simulink model "IFSSIM_Powertrain"  (R2025b)
settings: Solver=ode1  StartTime=0  StopTime=inf  FixedStep=0.0010416666666666671  RelTol=1e-3
undefined symbols (not defined in the file or in its folder): battery_builder_rtmsupport, gcbh, IFSSIM_eta, IFSSIM_gr, IFSSIM_Ipk, IFSSIM_Pmax, IFSSIM_Preg, IFSSIM_Tmax, IFSSIM_Treg, IFSSIM_Ts, IFSSIM_wregen
libraries: IFSSIM_Battery_6p19s5m1x_lib x5, fl_lib x3, nesl_utility x3
settings Model: Creator=raulmoran  LastModifiedBy=raulmoran

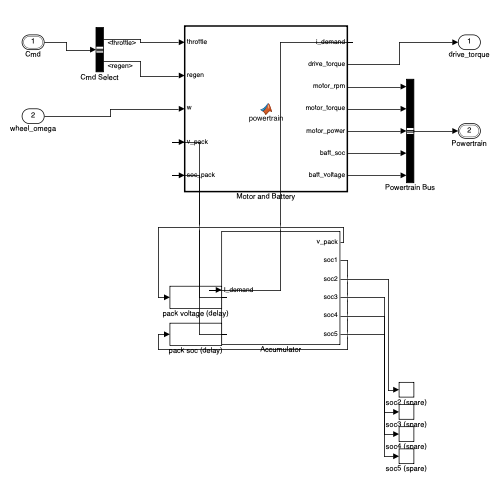
[thumbnail: Simulink's stored preview of the top-level diagram]
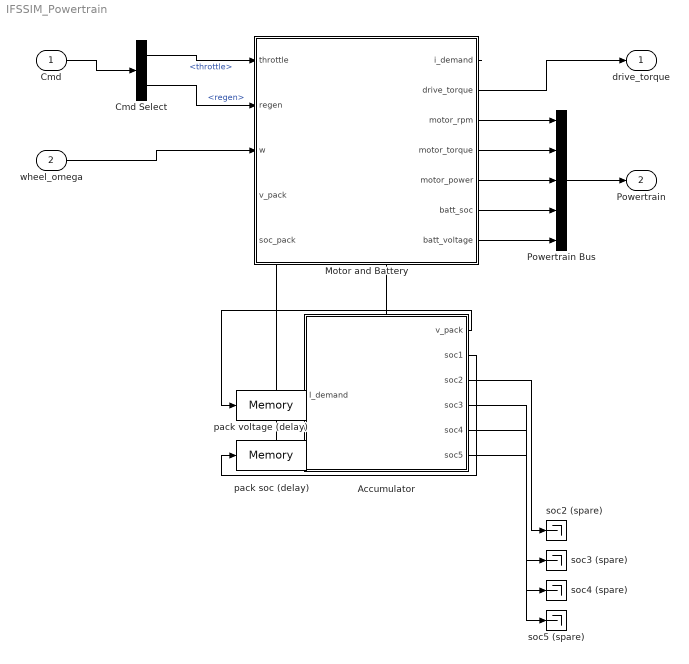
== system IFSSIM_Powertrain ==
  Cmd : Inport  OutDataTypeStr=Bus: IFSSIM_CmdBus  BusOutputAsStruct=on
  wheel_omega : Inport  Port=2  PortDimensions=4
  Accumulator : Subsystem
  Cmd Select : BusSelector  OutputSignals=throttle,regen
  Motor and Battery : MATLAB Function  TreatAsAtomicUnit=on
  Powertrain Bus : BusCreator  Inputs=5  OutDataTypeStr=Bus: IFSSIM_PowertrainBus  NonVirtualBus=on
  pack soc (delay) : Memory  InitialCondition=1
  pack voltage (delay) : Memory  InitialCondition=399
  soc2 (spare) : Terminator
  soc3 (spare) : Terminator
  soc4 (spare) : Terminator
  soc5 (spare) : Terminator
  drive_torque : Outport  PortDimensions=4
  Powertrain : Outport  Port=2  OutDataTypeStr=Bus: IFSSIM_PowertrainBus
  wires:
  Cmd/1 -> Cmd Select/1
  Powertrain Bus/1 -> Powertrain/1
  Cmd Select/1 -> Motor and Battery/1(throttle)  "<throttle>"
  Cmd Select/2 -> Motor and Battery/2(regen)  "<regen>"
  wheel_omega/1 -> Motor and Battery/3(w)
  pack voltage (delay)/1 -> Motor and Battery/4(v_pack)
  Accumulator/2(soc1) -> pack soc (delay)/1
  pack soc (delay)/1 -> Motor and Battery/5(soc_pack)
  Motor and Battery/1(i_demand) -> Accumulator/1(I_demand)
  Accumulator/1(v_pack) -> pack voltage (delay)/1
  Accumulator/3(soc2) -> soc2 (spare)/1
  Accumulator/4(soc3) -> soc3 (spare)/1
  Accumulator/5(soc4) -> soc4 (spare)/1
  Accumulator/6(soc5) -> soc5 (spare)/1
  Motor and Battery/2(drive_torque) -> drive_torque/1
  Motor and Battery/3(motor_rpm) -> Powertrain Bus/1
  Motor and Battery/4(motor_torque) -> Powertrain Bus/2
  Motor and Battery/5(motor_power) -> Powertrain Bus/3
  Motor and Battery/6(batt_soc) -> Powertrain Bus/4
  Motor and Battery/7(batt_voltage) -> Powertrain Bus/5

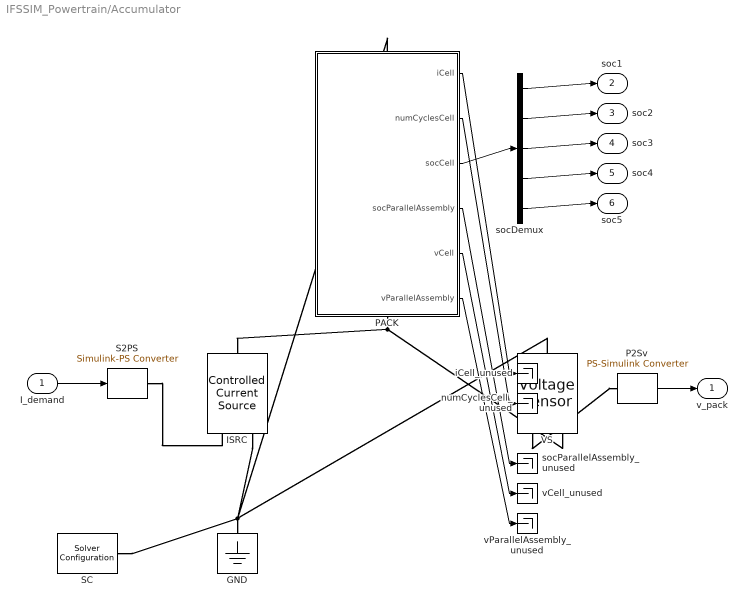
== system IFSSIM_Powertrain/Accumulator ==
  I_demand : Inport
  GND : fl_lib/Electrical/Electrical Elements/Electrical Reference
  ISRC : fl_lib/Electrical/Electrical Sources/Controlled Current Source
  P2Sv : nesl_utility/PS-Simulink Converter  PhysicalDomain=network_engine_domain  SubClassName=ps_output  LeftPortType=input  RightPortType=output  PseudoPeriodic=off  Frequencies=[]  VectorFormat=inherit  Unit=inherit  AffineConversion=off
  PACK : Subsystem  LoadFcn=battery_builder_rtmsupport('loadfcn',gcbh);
      settings: CopyFcn=battery_builder_rtmsupport('copyfcn',gcbh);  PreCopyFcn=battery_builder_rtmsupport('precopyfcn',gcbh);  PreDeleteFcn=battery_builder_rtmsupport('predeletefcn',gcbh);  PortSchema="{\"entries\":[{\"content\":{\"sides\":[{\"content\":{\"connectorIds\":[\"LConn1\"]},\"type\":\"ConnectorPlacement.EquallySpacedRectSide\",\"uuid\":\"b330ec76-9e31-4dfa-bf05-139a2ef62fc0\"},{\"content\":{\"connectorIds\":[\"RConn1\"],\"side\":\"RIGHT\"},\"type\":\"ConnectorPlacement.EquallySpacedRectSide\",\"uuid\":\"22fc76fa-e36b-473d-837a-d83c27c7e7c0\"},{\"content\":{\"side\":\"TOP\"},\"type\":\"ConnectorPlacement.EquallySpacedRectSide\",\"uuid\":\"ef8ee960-66ac-46a8-8763-1d10a91ef971\"},{\"content\":{\"connectorIds\":[\"Out1\",\"Out2\",\"Out3\",\"Out4\",\"Out5\",\"Out6\"],\"side\":\"BOTTOM\"},\"type\":\"ConnectorPlacement.EquallySpacedRectSide\",\"uuid\":\"8d6ec750-e234-47dd-8a49-b7b6d4e41f0f\"}]},\"type\":\"ConnectorPlacement.EquallySpacedConnector\",\"uuid\":\"b3d2af31-3e22-42b2-aab0-7b6ae654f145\"}],\"packageUris\":[\"http://schema.mathworks.com/mf0/Connector/R2020b\"],\"version\":\"1.0\"}"
      mask Display: image('$imagefile')
  S2PS : nesl_utility/Simulink-PS Converter  PhysicalDomain=network_engine_domain  SubClassName=ps_input  LeftPortType=input  RightPortType=output  PseudoPeriodic=off  Frequencies=[]  NoiseDistribution=none  NoiseParameters=[]  Unit=1  AffineConversion=off  FilteringAndDerivatives=provide  SimscapeFilterOrder=1  InputFilterTimeConstant=0.001  UdotUserProvided=0
  SC : nesl_utility/Solver Configuration  PhysicalDomain=network_engine_domain  SubClassName=solver  LeftPortType=input  RightPortType=generic  Tones=[]  Harmonics=[]  SimulateNoise=off  Profile=off  UseLocalSampling=off  EnableSwitchedLinearOptims=on  FrequencyDomain=off  UseCCode=off  RelTol=0.001  AbsTol=0.001  MinStep=1e-09  ToWorkspace=off  RevertToSquareIcSolve=off  NumHomotopyIterations=100  PhasorMode=off  PhasorModeNumHarmonics=1  ConsistencySolver=NEWTON_XTOL_AFTER_FTOL  IndexReductionMethod=DerivativeReplacement  DoDC=off  ResidualTolerance=1e-09  ConsistencyTolSource=GLOBAL  ConsistencyAbsTol=0.001  ConsistencyRelTol=0.001  ConsistencyTolFactor=0.001  UseLocalSolver=on  LocalSolverChoice=NE_BACKWARD_EULER_ADVANCER  ResolveIndetEquations=on  FunctionEvalNumThread=1  LocalSolverSampleTime=0.0010416666666666671  DoFixedCost=on  MaxNonlinIter=3  MaxModeIter=2  ComputeImpulses=off  ImpulseIterations=2  LinearAlgebra=auto  LinearAlgebraNumThread=0  EquationFormulation=NE_TIME_EF  DelaysMemoryBudget=1024  AutomaticFiltering=on  FilteringTimeConstant=0.001  PartitionStorageMethod=AS_NEEDED  PartitionMemoryBudget=1024  PartitionMethod=ROBUST  MultibodyUseLocalSolver=off  MultibodyLocalSolverChoice=ODE1  MultibodyLocalSolverSampleTime=0.001
  VS : fl_lib/Electrical/Electrical Sensors/Voltage Sensor
  iCell_unused : Terminator
  numCyclesCell_unused : Terminator
  socDemux : Demux  Outputs=5
  socParallelAssembly_unused : Terminator
  vCell_unused : Terminator
  vParallelAssembly_unused : Terminator
  v_pack : Outport
  soc1 : Outport  Port=2
  soc2 : Outport  Port=3
  soc3 : Outport  Port=4
  soc4 : Outport  Port=5
  soc5 : Outport  Port=6
  wires:
  I_demand/1 -> S2PS/1
  P2Sv/1 -> v_pack/1
  PACK/1(iCell) -> iCell_unused/1
  PACK/2(numCyclesCell) -> numCyclesCell_unused/1
  PACK/3(socCell) -> socDemux/1
  socDemux/1 -> soc1/1
  socDemux/2 -> soc2/1
  socDemux/3 -> soc3/1
  socDemux/4 -> soc4/1
  socDemux/5 -> soc5/1
  PACK/4(socParallelAssembly) -> socParallelAssembly_unused/1
  PACK/5(vCell) -> vCell_unused/1
  PACK/6(vParallelAssembly) -> vParallelAssembly_unused/1
  connections:
  S2PS/RConn1 -- ISRC/RConn1
  PACK/LConn1 -- ISRC/RConn2 -- VS/LConn1 -- GND/LConn1 -- SC/RConn1
  ISRC/LConn1 -- PACK/RConn1 -- VS/RConn2
  VS/RConn1 -- P2Sv/LConn1

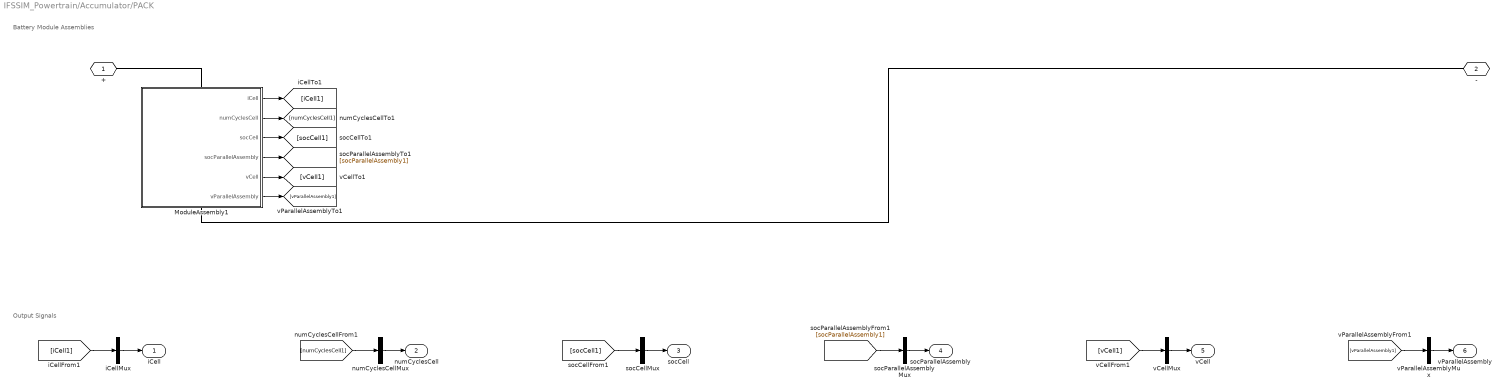
== system IFSSIM_Powertrain/Accumulator/PACK ==
  note: Output Signals
  note: Battery Module Assemblies
  ModuleAssembly1 : Subsystem  LoadFcn=battery_builder_rtmsupport('loadfcn',gcbh);
      settings: CopyFcn=battery_builder_rtmsupport('copyfcn',gcbh);  PreCopyFcn=battery_builder_rtmsupport('precopyfcn',gcbh);  PreDeleteFcn=battery_builder_rtmsupport('predeletefcn',gcbh);  PortSchema="{\"entries\":[{\"content\":{\"sides\":[{\"content\":{\"connectorIds\":[\"LConn1\"]},\"type\":\"ConnectorPlacement.EquallySpacedRectSide\",\"uuid\":\"b330ec76-9e31-4dfa-bf05-139a2ef62fc0\"},{\"content\":{\"connectorIds\":[\"RConn1\"],\"side\":\"RIGHT\"},\"type\":\"ConnectorPlacement.EquallySpacedRectSide\",\"uuid\":\"22fc76fa-e36b-473d-837a-d83c27c7e7c0\"},{\"content\":{\"side\":\"TOP\"},\"type\":\"ConnectorPlacement.EquallySpacedRectSide\",\"uuid\":\"ef8ee960-66ac-46a8-8763-1d10a91ef971\"},{\"content\":{\"connectorIds\":[\"Out1\",\"Out2\",\"Out3\",\"Out4\",\"Out5\",\"Out6\"],\"side\":\"BOTTOM\"},\"type\":\"ConnectorPlacement.EquallySpacedRectSide\",\"uuid\":\"c09a59a9-4f09-4d86-bb11-9b9750489816\"}]},\"type\":\"ConnectorPlacement.EquallySpacedConnector\",\"uuid\":\"b3d2af31-3e22-42b2-aab0-7b6ae654f145\"}],\"packageUris\":[\"http://schema.mathworks.com/mf0/Connector/R2020b\"],\"version\":\"1.0\"}"
      mask Display: image('$imagefile')
  iCellMux : Mux  Inputs=1
  numCyclesCellMux : Mux  Inputs=1
  socCellMux : Mux  Inputs=1
  socParallelAssemblyMux : Mux  Inputs=1
  vCellMux : Mux  Inputs=1
  vParallelAssemblyMux : Mux  Inputs=1
  + : PMIOPort  Side=Left
  - : PMIOPort  Port=2  Side=Right
  iCell : Outport
  numCyclesCell : Outport  Port=2
  socCell : Outport  Port=3
  socParallelAssembly : Outport  Port=4
  vCell : Outport  Port=5
  vParallelAssembly : Outport  Port=6
  wires:
  [vParallelAssembly1] -> vParallelAssemblyMux/1
  vParallelAssemblyMux/1 -> vParallelAssembly/1
  ModuleAssembly1/6(vParallelAssembly) -> [vParallelAssembly1]
  [vCell1] -> vCellMux/1
  vCellMux/1 -> vCell/1
  ModuleAssembly1/5(vCell) -> [vCell1]
  [socParallelAssembly1] -> socParallelAssemblyMux/1
  socParallelAssemblyMux/1 -> socParallelAssembly/1
  ModuleAssembly1/4(socParallelAssembly) -> [socParallelAssembly1]
  [socCell1] -> socCellMux/1
  socCellMux/1 -> socCell/1
  ModuleAssembly1/3(socCell) -> [socCell1]
  [numCyclesCell1] -> numCyclesCellMux/1
  numCyclesCellMux/1 -> numCyclesCell/1
  ModuleAssembly1/2(numCyclesCell) -> [numCyclesCell1]
  [iCell1] -> iCellMux/1
  iCellMux/1 -> iCell/1
  ModuleAssembly1/1(iCell) -> [iCell1]
  connections:
  ModuleAssembly1/RConn1 -- -/RConn1
  ModuleAssembly1/LConn1 -- +/RConn1

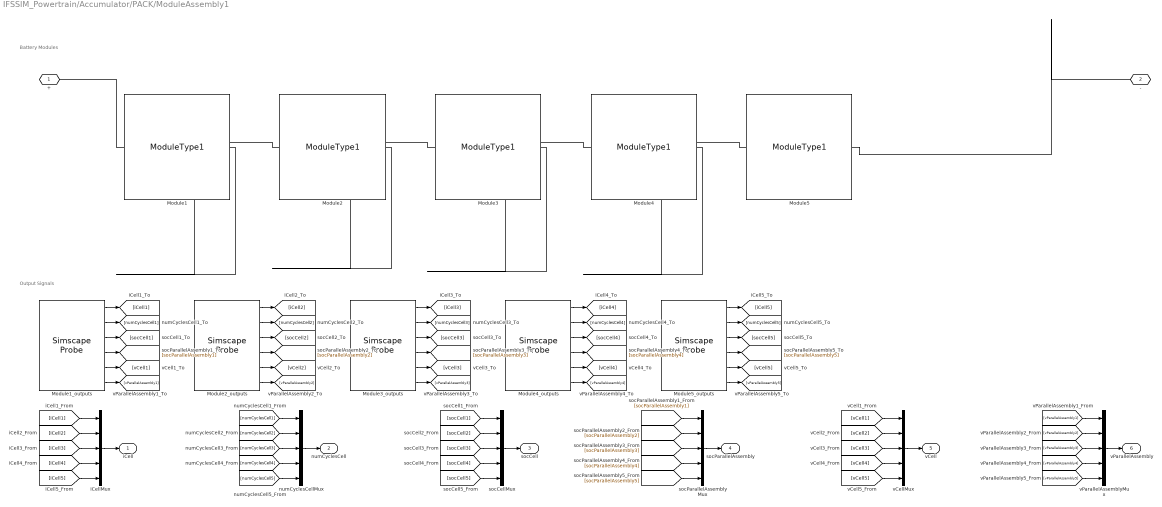
== system IFSSIM_Powertrain/Accumulator/PACK/ModuleAssembly1 ==
  note: Battery Modules
  note: Output Signals
  Module{1..5} (5 alike) : IFSSIM_Battery_6p19s5m1x_lib/Modules/ModuleType1  SOC_vecCell=IFSSIM_cell_SOC  V0_vecCell=IFSSIM_cell_V0 V  V_rangeCell=[0, inf] V  R0_vecCell=IFSSIM_cell_R0 Ohm  AHCell=IFSSIM_cell_AH A*hr  extrapolation_optionCell=simscape.enum.extrapolation.nearest  P=6  S=19  iCell_specify=off  iCell_priority=None  iCell=0 A  iCell_nominal_specify=off  iCell_nominal_value=1  iCell_nominal_unit=A  vCell_specify=off  vCell_priority=None  vCell=0 V  vCell_nominal_specify=off  vCell_nominal_value=1  vCell_nominal_unit=V  socCell_specify=on  socCell_priority=High  socCell=IFSSIM_SoC0  socCell_nominal_specify=off  socCell_nominal_value=1  socCell_nominal_unit=1  numCyclesCell_specify=off  numCyclesCell_priority=High  numCyclesCell=0  numCyclesCell_nominal_specify=off  numCyclesCell_nominal_value=1  numCyclesCell_nominal_unit=1  vParallelAssembly_specify=off  vParallelAssembly_priority=None  vParallelAssembly=repmat(0, 19, 1) V  vParallelAssembly_nominal_specify=off  vParallelAssembly_nominal_value=1  vParallelAssembly_nominal_unit=V  socParallelAssembly_specify=off  socParallelAssembly_priority=None  socParallelAssembly=repmat(1, 19, 1)  socParallelAssembly_nominal_specify=off  socParallelAssembly_nominal_value=1  socParallelAssembly_nominal_unit=1
      settings: InternalSimscapePortConfiguration="{\"Bottom\":[{\"id\":\"n\",\"label\":\"-\",\"type\":\"foundation.electrical.electrical\"}],\"Left\":[],\"Right\":[],\"Top\":[{\"id\":\"p\",\"label\":\"+\",\"type\":\"foundation.electrical.electrical\"}]}"
  Module1_outputs : SimscapeProbe  BoundBlock=10  Variables="{\"iCell\":{\"Probing\":\"ON\"},\"numCyclesCell\":{\"Probing\":\"ON\"},\"socCell\":{\"Probing\":\"ON\"},\"socParallelAssembly\":{\"Probing\":\"ON\"},\"vCell\":{\"Probing\":\"ON\"},\"vParallelAssembly\":{\"Probing\":\"ON\"}}"
  Module2_outputs : SimscapeProbe  BoundBlock=12  Variables="{\"iCell\":{\"Probing\":\"ON\"},\"numCyclesCell\":{\"Probing\":\"ON\"},\"socCell\":{\"Probing\":\"ON\"},\"socParallelAssembly\":{\"Probing\":\"ON\"},\"vCell\":{\"Probing\":\"ON\"},\"vParallelAssembly\":{\"Probing\":\"ON\"}}"
  Module3_outputs : SimscapeProbe  BoundBlock=14  Variables="{\"iCell\":{\"Probing\":\"ON\"},\"numCyclesCell\":{\"Probing\":\"ON\"},\"socCell\":{\"Probing\":\"ON\"},\"socParallelAssembly\":{\"Probing\":\"ON\"},\"vCell\":{\"Probing\":\"ON\"},\"vParallelAssembly\":{\"Probing\":\"ON\"}}"
  Module4_outputs : SimscapeProbe  BoundBlock=16  Variables="{\"iCell\":{\"Probing\":\"ON\"},\"numCyclesCell\":{\"Probing\":\"ON\"},\"socCell\":{\"Probing\":\"ON\"},\"socParallelAssembly\":{\"Probing\":\"ON\"},\"vCell\":{\"Probing\":\"ON\"},\"vParallelAssembly\":{\"Probing\":\"ON\"}}"
  Module5_outputs : SimscapeProbe  BoundBlock=18  Variables="{\"iCell\":{\"Probing\":\"ON\"},\"numCyclesCell\":{\"Probing\":\"ON\"},\"socCell\":{\"Probing\":\"ON\"},\"socParallelAssembly\":{\"Probing\":\"ON\"},\"vCell\":{\"Probing\":\"ON\"},\"vParallelAssembly\":{\"Probing\":\"ON\"}}"
  iCellMux : Mux  Inputs=5
  numCyclesCellMux : Mux  Inputs=5
  socCellMux : Mux  Inputs=5
  socParallelAssemblyMux : Mux  Inputs=5
  vCellMux : Mux  Inputs=5
  vParallelAssemblyMux : Mux  Inputs=5
  + : PMIOPort  Side=Left
  - : PMIOPort  Port=2  Side=Right
  iCell : Outport
  numCyclesCell : Outport  Port=2
  socCell : Outport  Port=3
  socParallelAssembly : Outport  Port=4
  vCell : Outport  Port=5
  vParallelAssembly : Outport  Port=6
  wires:
  Module1_outputs/1 -> [iCell1]
  iCellMux/1 -> iCell/1
  [iCell1] -> iCellMux/1
  Module1_outputs/2 -> [numCyclesCell1]
  numCyclesCellMux/1 -> numCyclesCell/1
  [numCyclesCell1] -> numCyclesCellMux/1
  Module1_outputs/3 -> [socCell1]
  socCellMux/1 -> socCell/1
  [socCell1] -> socCellMux/1
  Module1_outputs/4 -> [socParallelAssembly1]
  socParallelAssemblyMux/1 -> socParallelAssembly/1
  [socParallelAssembly1] -> socParallelAssemblyMux/1
  Module1_outputs/5 -> [vCell1]
  vCellMux/1 -> vCell/1
  [vCell1] -> vCellMux/1
  Module1_outputs/6 -> [vParallelAssembly1]
  vParallelAssemblyMux/1 -> vParallelAssembly/1
  [vParallelAssembly1] -> vParallelAssemblyMux/1
  Module2_outputs/1 -> [iCell2]
  [iCell2] -> iCellMux/2
  Module2_outputs/2 -> [numCyclesCell2]
  [numCyclesCell2] -> numCyclesCellMux/2
  Module2_outputs/3 -> [socCell2]
  [socCell2] -> socCellMux/2
  Module2_outputs/4 -> [socParallelAssembly2]
  [socParallelAssembly2] -> socParallelAssemblyMux/2
  Module2_outputs/5 -> [vCell2]
  [vCell2] -> vCellMux/2
  Module2_outputs/6 -> [vParallelAssembly2]
  [vParallelAssembly2] -> vParallelAssemblyMux/2
  Module3_outputs/1 -> [iCell3]
  [iCell3] -> iCellMux/3
  Module3_outputs/2 -> [numCyclesCell3]
  [numCyclesCell3] -> numCyclesCellMux/3
  Module3_outputs/3 -> [socCell3]
  [socCell3] -> socCellMux/3
  Module3_outputs/4 -> [socParallelAssembly3]
  [socParallelAssembly3] -> socParallelAssemblyMux/3
  Module3_outputs/5 -> [vCell3]
  [vCell3] -> vCellMux/3
  Module3_outputs/6 -> [vParallelAssembly3]
  [vParallelAssembly3] -> vParallelAssemblyMux/3
  Module4_outputs/1 -> [iCell4]
  [iCell4] -> iCellMux/4
  Module4_outputs/2 -> [numCyclesCell4]
  [numCyclesCell4] -> numCyclesCellMux/4
  Module4_outputs/3 -> [socCell4]
  [socCell4] -> socCellMux/4
  Module4_outputs/4 -> [socParallelAssembly4]
  [socParallelAssembly4] -> socParallelAssemblyMux/4
  Module4_outputs/5 -> [vCell4]
  [vCell4] -> vCellMux/4
  Module4_outputs/6 -> [vParallelAssembly4]
  [vParallelAssembly4] -> vParallelAssemblyMux/4
  Module5_outputs/1 -> [iCell5]
  [iCell5] -> iCellMux/5
  Module5_outputs/2 -> [numCyclesCell5]
  [numCyclesCell5] -> numCyclesCellMux/5
  Module5_outputs/3 -> [socCell5]
  [socCell5] -> socCellMux/5
  Module5_outputs/4 -> [socParallelAssembly5]
  [socParallelAssembly5] -> socParallelAssemblyMux/5
  Module5_outputs/5 -> [vCell5]
  [vCell5] -> vCellMux/5
  Module5_outputs/6 -> [vParallelAssembly5]
  [vParallelAssembly5] -> vParallelAssemblyMux/5
  connections:
  Module2/LConn1 -- Module1/RConn1
  Module3/LConn1 -- Module2/RConn1
  Module4/LConn1 -- Module3/RConn1
  Module5/LConn1 -- Module4/RConn1
  Module1/LConn1 -- +/RConn1
  Module5/RConn1 -- -/RConn1

== matlab function IFSSIM_Powertrain/Motor and Battery ==
  data: throttle input size=1; i_demand output size=1; regen input size=1; w input size=4; v_pack input size=1; soc_pack input size=1; drive_torque output size=4; motor_rpm output size=1; motor_torque output size=1; motor_power output size=1; batt_soc output size=1; batt_voltage output size=1; IFSSIM_Ts parameter size=1; IFSSIM_gr parameter size=1; IFSSIM_eta parameter size=1; IFSSIM_Tmax parameter size=1; IFSSIM_Pmax parameter size=1; IFSSIM_Treg parameter size=1; IFSSIM_Preg parameter size=1; IFSSIM_Ipk parameter size=1; IFSSIM_wregen parameter size=1
function [i_demand, drive_torque, motor_rpm, motor_torque, motor_power, batt_soc, batt_voltage] = ...
         powertrain(throttle, regen, w, v_pack, soc_pack, IFSSIM_Ts, IFSSIM_gr, IFSSIM_eta, IFSSIM_Tmax, IFSSIM_Pmax, IFSSIM_Treg, IFSSIM_Preg, IFSSIM_Ipk, IFSSIM_wregen)
%#codegen
% Motor envelope, single-speed drivetrain, battery state of charge.
%
% Wheel order FL, FR, RL, RR.

Ts = IFSSIM_Ts;

% TORQUE SPLIT. RWD today. Change this vector to try in-wheel motors or torque
% vectoring — it is written out precisely so that experiment cannot silently
% remain an RWD experiment.
split = [0; 0; 0.5; 0.5];

% Motor speed follows the DRIVEN wheels through the single reduction. Using the
% mean of the driven pair is the open-differential assumption; a spool or an LSD
% would change this and so would per-wheel motors.
driven = split > 0;
if any(driven)
    w_drv = sum(w .* driven) / sum(driven);
else
    w_drv = 0;
end
w_motor = w_drv * IFSSIM_gr;                 % rad/s
motor_rpm = w_motor * 60 / (2*pi);

% --- torque demand -------------------------------------------------
% Drive and regen are SUMMED. Chaos discards one of them: its wheel solver
% picks braking OR driving by magnitude, so a simultaneous regen-and-drive
% command loses a channel silently. Summing is what the real inverter does.
th = max(0, min(1, throttle));
rg = max(0, min(1, regen));
% REGEN OPPOSES MOTION; it does not create it. Written as a plain
% -rg*Treg, a regen command at rest is just reverse drive: the A/B harness
% caught the car reversing 17.8 m in 3 s at 9.9 m/s with regen 1.0 from a
% standstill, wheels turning backwards at -48.6 rad/s. There is no back-EMF
% from a stationary wheel and no kinetic energy to recover, so the torque
% must fade with speed.
%
% tanh, not sign, and for the reason the tyre block gives for the same
% choice: sign() chatters about zero every step at 1/960 s. This also means
% regen RESISTS motion but cannot HOLD a stopped car, which is correct -- it
% is a motor, not a parking brake, and this car has no service brake to
% stand in for one.
T_cmd = th*IFSSIM_Tmax - rg*IFSSIM_Treg*tanh(w_motor/IFSSIM_wregen);

% --- envelope --------------------------------------------------------
wa = max(abs(w_motor), 1e-3);

% WHAT THE ACCUMULATOR CAN ACTUALLY GIVE, at the voltage it is at right now
% rather than at its nameplate. This is the limit that did not exist before:
% the envelope was min(Tmax, Pmax/w), the battery was computed and ignored,
% and the plant handed out 80 kW from a pack that can supply 51.
%
% v_pack is last step's terminal voltage, so it already has the sag from the
% current we are about to ask for. Multiplied by what the pack can pass, it
% is the electrical power available -- and, the motor being lossless here
% (see 'electrical' below), the power available at the shaft.
vb     = max(v_pack, 1);
P_pack = vb * IFSSIM_Ipk;

if T_cmd >= 0
    P_avail = min(IFSSIM_Pmax, P_pack);
    T = min(T_cmd,  min(IFSSIM_Tmax, P_avail / wa));
else
    % REGEN IS POWER LIMITED LONG BEFORE IT IS TORQUE LIMITED. MaxRegenPower is
    % the cell input-current cap and at any real speed it binds first, by a
    % large factor. This is the whole reason the car cannot stop as hard as its
    % motor torque figure suggests.
    T = max(T_cmd, -min(IFSSIM_Treg, IFSSIM_Preg / wa));
end
motor_torque = T;

% --- electrical ------------------------------------------------------
% EFFICIENCY IS CHARGED ONCE, AT THE GEARS (below), and NOT here as well.
% This used to divide by eta here too, so pack-to-road was eta^2 = 0.846 --
% while the comment at the wheels claimed the double charge had been
% removed. DrivetrainEfficiency is sourced as the DRIVETRAIN ('workbook
% quotes 92-98%'), and every other model on the branch -- fs_track_cycle,
% endurance_current, vd_gg, pt_model -- charges it once between the pack
% and the road. So the motor and inverter are LOSSLESS in this block:
% electrical power equals shaft power. That is an assumption, not a fact;
% a sourced motor efficiency would be a separate parameter, charged here.
P_mech = T * w_motor;
P_elec = P_mech;
motor_power = P_elec;

% The battery is no longer modelled here. Open-circuit voltage, capacity,
% internal resistance and the state of charge all live in the Simscape
% accumulator now, which is five modules of real cells rather than a line
% through two voltages. What crosses this boundary is a CURRENT DEMAND out
% and a terminal voltage and state of charge back.
%
% Dividing by the terminal voltage rather than the open-circuit voltage is
% deliberate: the pack has already sagged under load, and the current needed
% to make a given power is set by the voltage actually present.
i_demand    = P_elec / vb;
batt_voltage = v_pack;
batt_soc     = soc_pack;

% --- to the wheels ---------------------------------------------------
% EFFICIENCY IS DIRECTIONAL, and it was not. The comment here used to read
% efficiency applies to the mechanical path in both directions, and the
% code multiplied by eta unconditionally, which is wrong in each direction
% for a different reason.
%
% Driving, the motor makes T and the wheel receives less: T*gr*eta. This is
% the ONE place eta is charged; the electrical branch above no longer
% charges it again (it did, and road power was eta^2 of pack power).
%
% Regenerating, the wheel drives the motor, so the wheel must supply the
% braking torque PLUS the losses: T*gr/eta, not T*gr*eta. Written the old
% way the wheel braked with less torque than the motor absorbed, which is
% energy appearing from nowhere. Wheel to pack is now eta exactly, once.
%
% split SUMS TO 1, so this distributes the total wheel torque. An earlier
% version multiplied by 2 as well, which handed each driven wheel the whole
% motor torque and doubled the car's acceleration. The stall test caught it.
if T >= 0
    T_wheel = T * IFSSIM_gr * IFSSIM_eta;      % losses reduce what arrives
else
    T_wheel = T * IFSSIM_gr / IFSSIM_eta;      % losses must also be braked
end
drive_torque = split * T_wheel;
end
